simulink model "Q4_W1"  (R2020b)
settings: Solver=VariableStepAuto  StartTime=0.0  StopTime=10.0  RelTol=1e-3
settings Model: Creator=hp  LastModifiedBy=hp

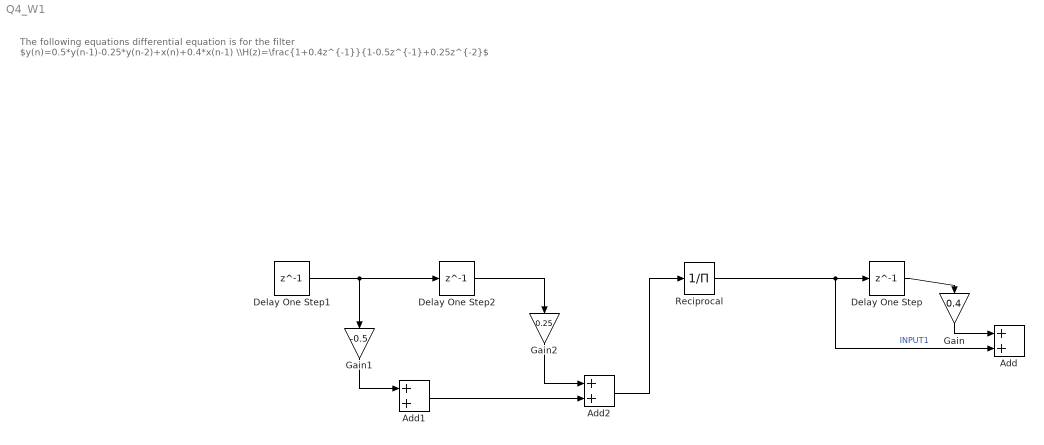
== system Q4_W1 ==
  note: The following equations differential equation is for the filter
      | $y(n)=0.5*y(n-1)-0.25*y(n-2)+x(n)+0.4*x(n-1) \\H(z)=\frac{1+0.4z^{-1}}{1-0.5z^{-1}+0.25z^{-2}$
  Add : Sum
  Add1 : Sum
  Add2 : Sum
  Delay One Step : Delay  DelayLength=1
  Delay One Step1 : Delay  DelayLength=1
  Delay One Step2 : Delay  DelayLength=1
  Gain : Gain  Gain=0.4
  Gain1 : Gain  Gain=-0.5
  Gain2 : Gain  Gain=0.25
  Reciprocal : Product  Inputs=/
  wires:
  Delay One Step/1 -> Gain/1
  Gain/1 -> Add/1
  Reciprocal/1 -> Add/2, Delay One Step/1  "INPUT1"
  Delay One Step1/1 -> Delay One Step2/1, Gain1/1
  Gain1/1 -> Add1/1
  ? -> Add1/2, Delay One Step1/1  "INPUT"
  Delay One Step2/1 -> Gain2/1
  Add1/1 -> Add2/2
  Gain2/1 -> Add2/1
  Add2/1 -> Reciprocal/1
